simulink model "useful_blocks"  (Simulink 5.0)
settings: Solver=ode45  StartTime=0.0  StopTime=10.0  RelTol=1e-3
undefined symbols (not defined in the file or in its folder): fs, get
libraries: dspxfrm3 x1, dspsrcs4 x1, dspsnks4 x1
settings Model: Creator=hvanhaut  LastModifiedBy=hvanhaut  ExtModeAutoUpdateStatusClock=off  BooleanDataType=off

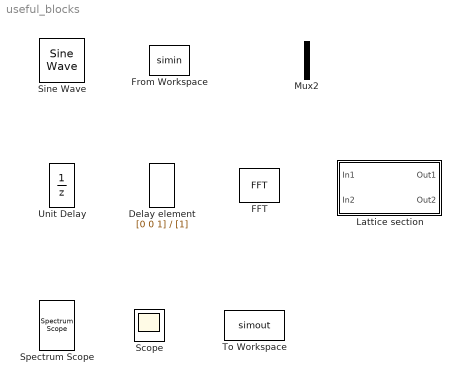
== system useful_blocks ==
  Delay element : DiscreteFilter  Numerator=[0 0 1]  Denominator=[1]  SampleTime=-1
  FFT : dspxfrm3/FFT  CompMethod=Table lookup  TableOpt=Speed  BitRevOrder=off
  From Workspace : FromWorkspace  VariableName=simin  SampleTime=1/fs  OutputAfterFinalValue=Holding final value
  Lattice section : Subsystem  mask{ts=-1, rc=1}
      mask prompts: ts "Sampling time (-1 for inherited):"; rc "Reflection coefficient:"
      mask help:
      | Section within the lattice representation of a FIR filter with a given reflection coefficient.
      | Click 'Look under mask' in the 'Edit' menu, or right-click on this block and choose 'Look under mask' to see what is underneath.
  Mux2 : Mux  Inputs=2
  Scope : Scope
  Sine Wave : dspsrcs4/Sine Wave  Amplitude=1  Frequency=25  Phase=0  SampleMode=Discrete  OutComplex=Real  CompMethod=Trigonometric fcn  TableSize=Speed  SampleTime=1/1000  SamplesPerFrame=1  dataType=double  wordLen=16  udDataType=sfix(16)  fracBitsMode=Best precision  numFracBits=14  ResetState=Restart at time zero
  Spectrum Scope : dspsnks4/Spectrum Scope  ScopeProperties=off  Domain=Frequency  HorizSpan=1  UseBuffer=on  BufferSize=512  Overlap=256  inpFftLenInherit=on  FFTlength=512  numAvg=2  DisplayProperties=off  AxisGrid=on  Memory=off  FrameNumber=on  AxisLegend=off  AxisZoom=off  OpenScopeAtSimStart=off  OpenScopeImmediately=off  FigPos=get(0,'defaultfigureposition')  AxisProperties=on  XUnits=Hertz  XRange=[0...Fs/2]  InheritXIncr=on  XIncr=1.0  XLabel=Samples  YUnits=dB  YLabel=Magnitude, dB  LineProperties=off
      settings: YMin=-127.040419076021  YMax=32.8248044573492
  To Workspace : ToWorkspace  VariableName=simout  SampleTime=-1  SaveFormat=Array
  Unit Delay : UnitDelay  SampleTime=-1

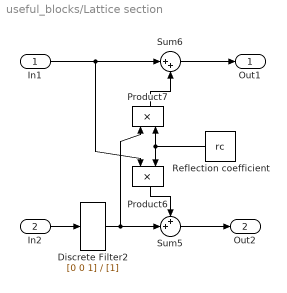
== system useful_blocks/Lattice section ==
  In1 : Inport
  In2 : Inport  Port=2
  Discrete Filter2 : DiscreteFilter  Numerator=[0 0 1]  Denominator=[1]  SampleTime=ts
  Product6 : Product  Orientation=down  SaturateOnIntegerOverflow=on  InputSameDT=on
  Product7 : Product  Orientation=up  SaturateOnIntegerOverflow=on  InputSameDT=on
  Reflection coefficient : Constant  Orientation=left  Value=rc
  Sum5 : Sum  Inputs=++|  InputSameDT=on
  Sum6 : Sum  Inputs=|++  InputSameDT=on
  Out1 : Outport
  Out2 : Outport  Port=2
  wires:
  Discrete Filter2/1 -> Product7/1, Sum5/2
  Product6/1 -> Sum5/1
  Product7/1 -> Sum6/2
  In1/1 -> Product6/1, Sum6/1
  In2/1 -> Discrete Filter2/1
  Sum6/1 -> Out1/1
  Sum5/1 -> Out2/1
  Reflection coefficient/1 -> Product7/2, Product6/2
